simulink model "acceleration_event_simulink"  (R2023b)
settings: Solver=VariableStepAuto  StartTime=0.0  StopTime=10.0  RelTol=1e-3
settings Model: Creator=bglen  LastModifiedBy=bglen
settings DebuggingCC: UnconnectedInputMsg=warning  UnconnectedOutputMsg=warning  UnconnectedLineMsg=warning
settings ModelReferenceCC: EnableRefExpFcnMdlSchedulingChecks=on
settings RTWCC: DLArmComputeVersion=19.05

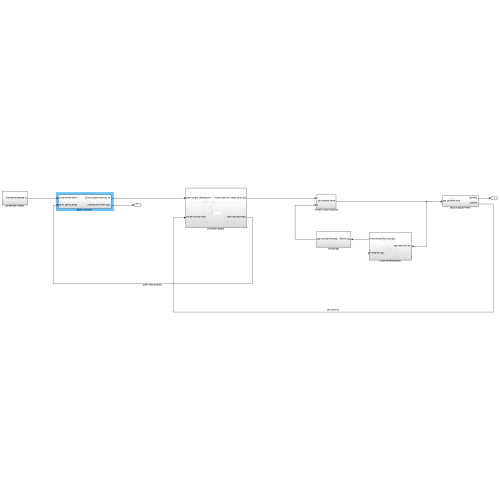
[thumbnail: Simulink's stored preview of the top-level diagram]
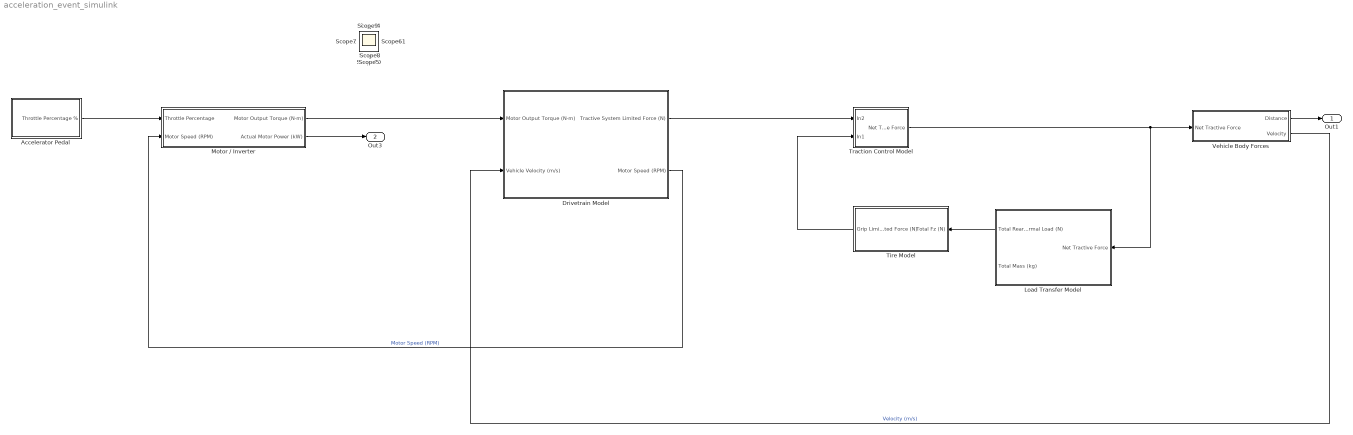
== system acceleration_event_simulink ==
  Accelerator Pedal : Subsystem
  Drivetrain Model : Subsystem
  Load Transfer Model : Subsystem
  Motor / Inverter : Subsystem
  Tire Model : Subsystem
  Traction Control Model : Subsystem
  Vehicle Body Forces : Subsystem
  Out1 : Outport
  Out3 : Outport  Port=2
  Scope{,1..11} (12 alike) : Scope
  wires:
  Load Transfer Model/1(Total Rear Normal Load (N)) -> Tire Model/1(Total Fz (N))
  Vehicle Body Forces/1(Distance) -> Out1/1
  Vehicle Body Forces/2(Velocity) -> Drivetrain Model/2(Vehicle Velocity (m/s))  "Velocity (m/s)"
  Traction Control Model/1(Net Tractive Force) -> Load Transfer Model/1(Net Tractive Force), Vehicle Body Forces/1(Net Tractive Force)
  Tire Model/1(Grip Limited Force (N)) -> Traction Control Model/2(In1)
  Drivetrain Model/1(Tractive System Limited Force (N)) -> Traction Control Model/1(In2)
  Drivetrain Model/2(Motor Speed (RPM)) -> Motor / Inverter/2(Motor Speed (RPM))  "Motor Speed (RPM)"
  Motor / Inverter/1(Motor Output Torque (N-m)) -> Drivetrain Model/1(Motor Output Torque (N-m))
  Motor / Inverter/2(Actual Motor Power (kW)) -> Out3/1
  Accelerator Pedal/1(Throttle Percentage %) -> Motor / Inverter/1(Throttle Percentage)

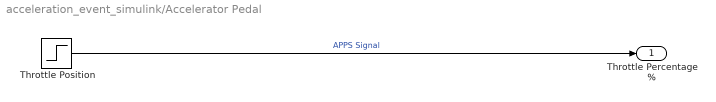
== system acceleration_event_simulink/Accelerator Pedal ==
  Throttle Position : Step  SampleTime=0
  Throttle Percentage % : Outport
  wires:
  Throttle Position/1 -> Throttle Percentage %/1  "APPS Signal"

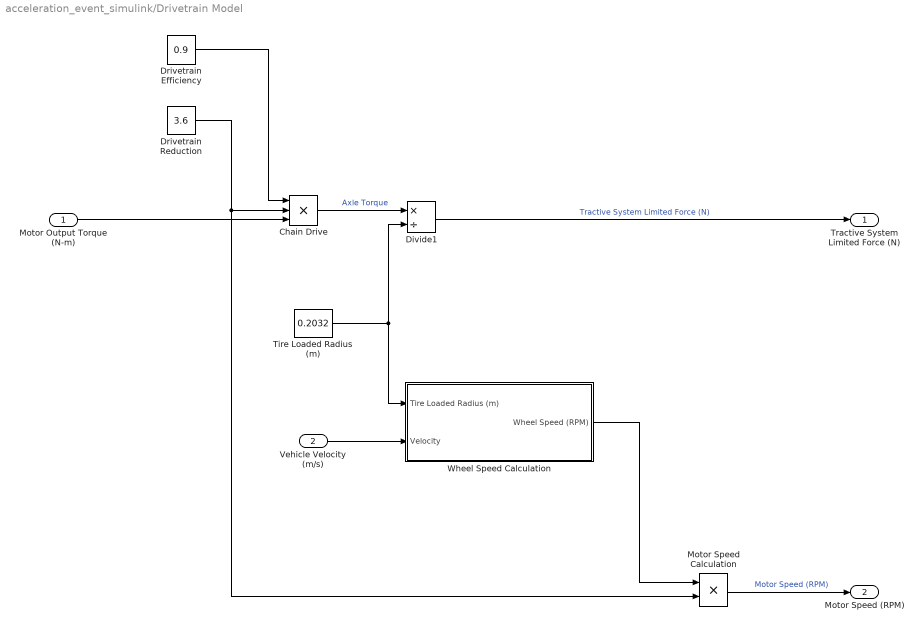
== system acceleration_event_simulink/Drivetrain Model ==
  Motor Output Torque (N-m) : Inport
  Vehicle Velocity (m/s) : Inport  Port=2
  "  Motor Speed Calculation" : Product
  Chain Drive : Product  Inputs=3
  Divide1 : Product  Inputs=*/
  Drivetrain Efficiency : Constant  Value=0.9
  Drivetrain Reduction : Constant  Value=3.6
  Tire Loaded Radius (m) : Constant  Value=0.2032
  Wheel Speed Calculation : Subsystem
  Tractive System Limited Force (N) : Outport
  Motor Speed (RPM) : Outport  Port=2
  wires:
  Divide1/1 -> Tractive System Limited Force (N)/1  "Tractive System Limited Force (N)"
  Tire Loaded Radius (m)/1 -> Wheel Speed Calculation/1(Tire Loaded Radius (m)), Divide1/2
  Chain Drive/1 -> Divide1/1  "Axle Torque"
  Motor Output Torque (N-m)/1 -> Chain Drive/3
  Drivetrain Efficiency/1 -> Chain Drive/1
  Drivetrain Reduction/1 -> "  Motor Speed Calculation"/2, Chain Drive/2
  Vehicle Velocity (m/s)/1 -> Wheel Speed Calculation/2(Velocity)
  Wheel Speed Calculation/1(Wheel Speed (RPM)) -> "  Motor Speed Calculation"/1
  "  Motor Speed Calculation"/1 -> Motor Speed (RPM)/1  "Motor Speed (RPM)"

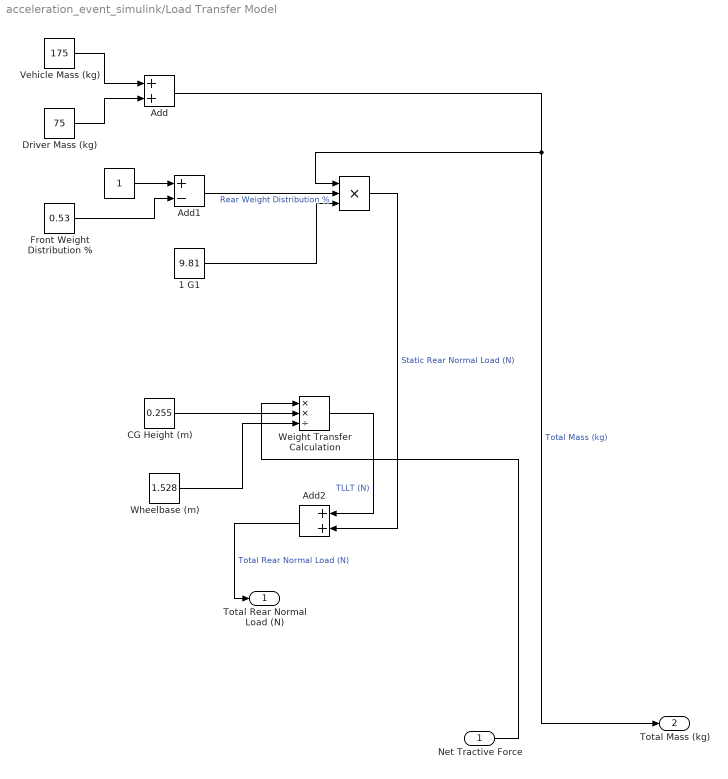
== system acceleration_event_simulink/Load Transfer Model ==
  Net Tractive Force : Inport
  " " : Constant
  "  " : Product  Inputs=3
  "  Weight Transfer Calculation" : Product  Inputs=**/
  1 G1 : Constant  Value=9.81
  Add : Sum
  Add1 : Sum  Inputs=+-
  Add2 : Sum
  CG Height (m) : Constant  Value=0.255
  Driver Mass (kg) : Constant  Value=75
  Front Weight Distribution % : Constant  Value=0.53
  Vehicle Mass (kg) : Constant  Value=175
  Wheelbase (m) : Constant  Value=1.528
  Total Rear Normal Load (N) : Outport
  Total Mass (kg) : Outport  Port=2
  wires:
  Net Tractive Force/1 -> "  Weight Transfer Calculation"/1
  " "/1 -> Add1/1
  "  "/1 -> Add2/2  "Static Rear Normal Load (N)"
  Add1/1 -> "  "/2  "Rear Weight Distribution %"
  Add2/1 -> Total Rear Normal Load (N)/1  "Total Rear Normal Load (N)"
  1 G1/1 -> "  "/3
  Vehicle Mass (kg)/1 -> Add/1
  CG Height (m)/1 -> "  Weight Transfer Calculation"/2
  Front Weight Distribution %/1 -> Add1/2
  Wheelbase (m)/1 -> "  Weight Transfer Calculation"/3
  "  Weight Transfer Calculation"/1 -> Add2/1  "TLLT (N)"
  Add/1 -> Total Mass (kg)/1, "  "/1  "Total Mass (kg)"
  Driver Mass (kg)/1 -> Add/2

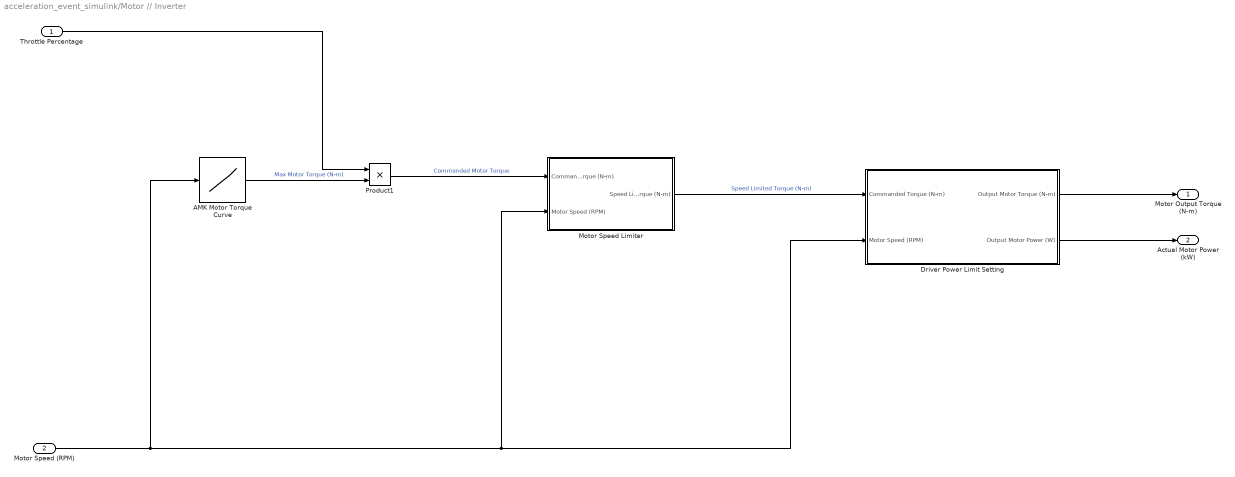
== system acceleration_event_simulink/Motor // Inverter ==
  Throttle Percentage : Inport
  Motor Speed (RPM) : Inport  Port=2
  AMK Motor Torque Curve : Lookup_n-D  NumberOfTableDimensions=1  BreakpointsForDimension1=[0;28.3870968;1447.74194;3179.35484;4740.64516;7267.09677;9055.48387;10872.2581;12178.0645;13029.6774;13994.8387;14846.4516;15612.9032;16095.4839;16805.1613;17571.6129;18423.2258;19274.8387;19785.8065;19984.5161]  Table=[21.31;21.3068182;21.3068182;21.3068182;21.3068182;21.3068182;21.3068182;21.3068182;21.3068182;21.3068182;21.3068182;21.3068182;21.3068182;20.9659091;19.9431818;18.5795455;17.0454545;15.3409091;14.1477273;13.6363636]  InternalRulePriority=Speed  RndMeth=Simplest
  Driver Power Limit Setting : Subsystem
  Motor Speed Limiter : Subsystem
  Product1 : Product
  Motor Output Torque (N-m) : Outport
  Actual Motor Power (kW) : Outport  Port=2
  wires:
  Throttle Percentage/1 -> Product1/1
  Product1/1 -> Motor Speed Limiter/1(Commanded Torque (N-m))  "Commanded Motor Torque"
  Motor Speed (RPM)/1 -> Motor Speed Limiter/2(Motor Speed (RPM)), Driver Power Limit Setting/2(Motor Speed (RPM)), AMK Motor Torque Curve/1
  AMK Motor Torque Curve/1 -> Product1/2  "Max Motor Torque (N-m)"
  Motor Speed Limiter/1(Speed Limited Motor Torque (N-m)) -> Driver Power Limit Setting/1(Commanded Torque (N-m))  "Speed Limited Torque (N-m)"
  Driver Power Limit Setting/1(Output Motor Torque (N-m)) -> Motor Output Torque (N-m)/1
  Driver Power Limit Setting/2(Output Motor Power (W)) -> Actual Motor Power (kW)/1

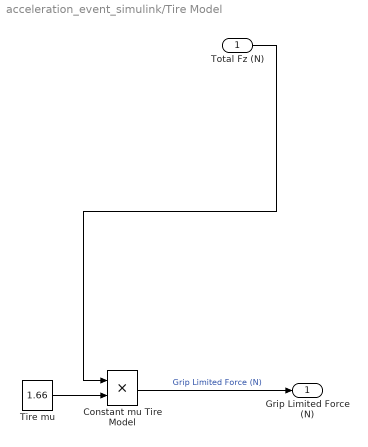
== system acceleration_event_simulink/Tire Model ==
  Total Fz (N) : Inport
  Constant mu Tire Model : Product
  Tire mu : Constant  Value=1.66
  Grip Limited Force (N) : Outport
  wires:
  Total Fz (N)/1 -> Constant mu Tire Model/1
  Constant mu Tire Model/1 -> Grip Limited Force (N)/1  "Grip Limited Force (N)"
  Tire mu/1 -> Constant mu Tire Model/2

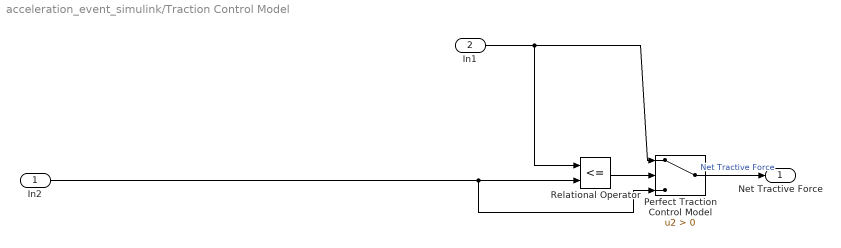
== system acceleration_event_simulink/Traction Control Model ==
  In2 : Inport
  In1 : Inport  Port=2
  Perfect Traction Control Model : Switch  Criteria=u2 > Threshold  SaturateOnIntegerOverflow=off  InputSameDT=off
  Relational Operator : RelationalOperator  Operator=<=  OutDataTypeStr=boolean  RndMeth=Simplest  InputSameDT=off
  Net Tractive Force : Outport
  wires:
  Perfect Traction Control Model/1 -> Net Tractive Force/1  "Net Tractive Force"
  Relational Operator/1 -> Perfect Traction Control Model/2
  In1/1 -> Relational Operator/1, Perfect Traction Control Model/1
  In2/1 -> Perfect Traction Control Model/3, Relational Operator/2

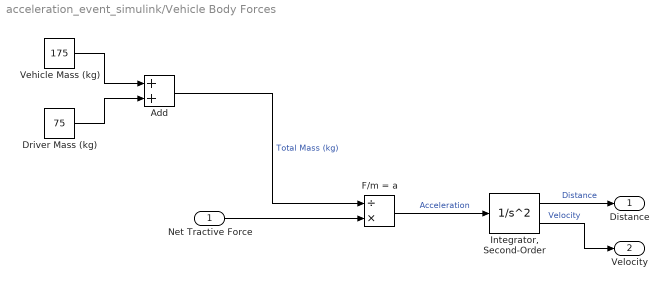
== system acceleration_event_simulink/Vehicle Body Forces ==
  Net Tractive Force : Inport
  Add : Sum
  Driver Mass (kg) : Constant  Value=75
  F/m = a : Product  Inputs=/*
  "Integrator, Second-Order" : SecondOrderIntegrator  LimitX=on  UpperLimitX=75
  Vehicle Mass (kg) : Constant  Value=175
  Distance : Outport
  Velocity : Outport  Port=2
  wires:
  "Integrator, Second-Order"/2 -> Velocity/1  "Velocity"
  Net Tractive Force/1 -> F/m = a/2
  "Integrator, Second-Order"/1 -> Distance/1  "Distance"
  F/m = a/1 -> "Integrator, Second-Order"/1  "Acceleration"
  Driver Mass (kg)/1 -> Add/2
  Vehicle Mass (kg)/1 -> Add/1
  Add/1 -> F/m = a/1  "Total Mass (kg)"

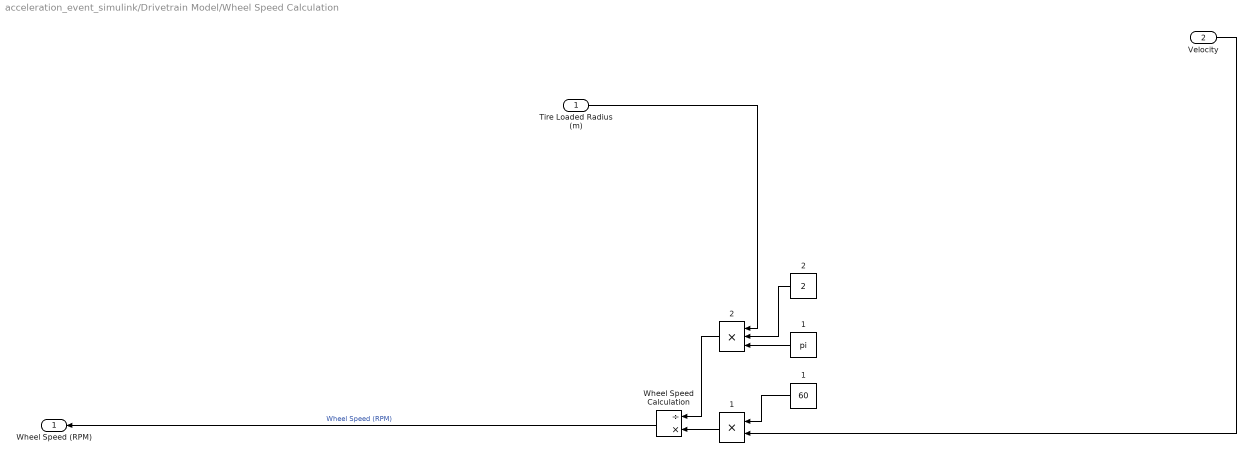
== system acceleration_event_simulink/Drivetrain Model/Wheel Speed Calculation ==
  Tire Loaded Radius (m) : Inport
  Velocity : Inport  Port=2
  "  1" : Product
  "  2" : Product  Inputs=3
  " 1" : Constant  Value=60
  1 : Constant  Value=pi
  2 : Constant  Value=2
  Wheel Speed Calculation : Product  Inputs=/*
  Wheel Speed (RPM) : Outport
  wires:
  Tire Loaded Radius (m)/1 -> "  2"/1
  Velocity/1 -> "  1"/2
  " 1"/1 -> "  1"/1
  "  2"/1 -> Wheel Speed Calculation/1
  1/1 -> "  2"/3
  "  1"/1 -> Wheel Speed Calculation/2
  Wheel Speed Calculation/1 -> Wheel Speed (RPM)/1  "Wheel Speed (RPM)"
  2/1 -> "  2"/2

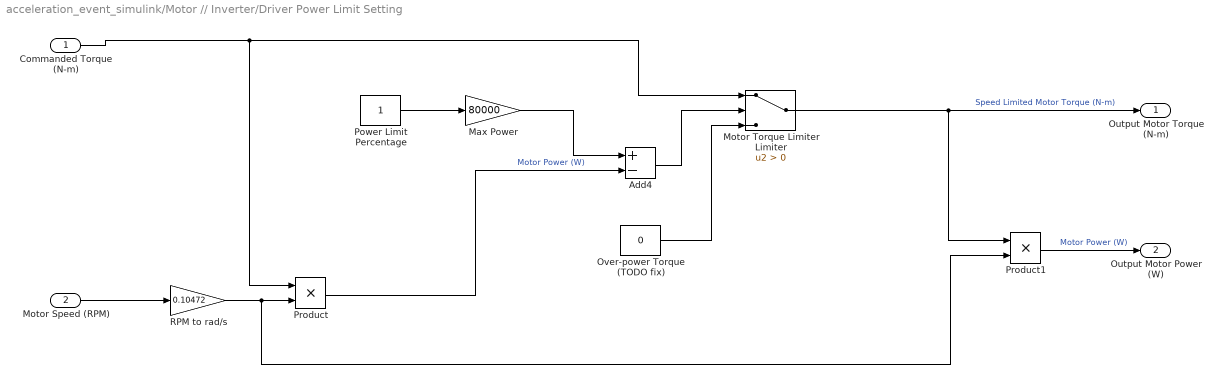
== system acceleration_event_simulink/Motor // Inverter/Driver Power Limit Setting ==
  Commanded Torque (N-m) : Inport
  Motor Speed (RPM) : Inport  Port=2
  Add4 : Sum  Inputs=+-
  Max Power : Gain  Gain=80000
  Motor Torque Limiter Limiter : Switch  Criteria=u2 > Threshold  SaturateOnIntegerOverflow=off  InputSameDT=off
  Over-power Torque (TODO fix) : Constant  Value=0
  Power Limit Percentage : Constant
  Product : Product
  Product1 : Product
  RPM to rad/s : Gain  Gain=0.10472
  Output Motor Torque (N-m) : Outport
  Output Motor Power (W) : Outport  Port=2
  wires:
  Add4/1 -> Motor Torque Limiter Limiter/2
  Commanded Torque (N-m)/1 -> Motor Torque Limiter Limiter/1, Product/1
  Motor Torque Limiter Limiter/1 -> Product1/1, Output Motor Torque (N-m)/1  "Speed Limited Motor Torque (N-m)"
  Over-power Torque (TODO fix)/1 -> Motor Torque Limiter Limiter/3
  Motor Speed (RPM)/1 -> RPM to rad/s/1
  Power Limit Percentage/1 -> Max Power/1
  Product/1 -> Add4/2  "Motor Power (W)"
  Max Power/1 -> Add4/1
  RPM to rad/s/1 -> Product1/2, Product/2
  Product1/1 -> Output Motor Power (W)/1  "Motor Power (W)"

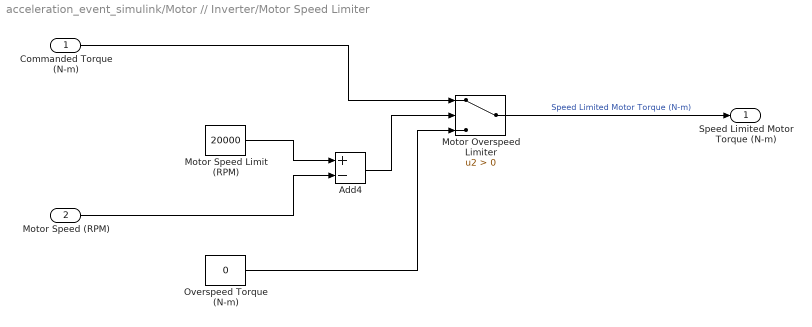
== system acceleration_event_simulink/Motor // Inverter/Motor Speed Limiter ==
  Commanded Torque (N-m) : Inport
  Motor Speed (RPM) : Inport  Port=2
  Add4 : Sum  Inputs=+-
  Motor Overspeed Limiter : Switch  Criteria=u2 > Threshold  SaturateOnIntegerOverflow=off  InputSameDT=off
  Motor Speed Limit (RPM) : Constant  Value=20000
  Overspeed Torque (N-m) : Constant  Value=0
  Speed Limited Motor Torque (N-m) : Outport
  wires:
  Motor Speed (RPM)/1 -> Add4/2
  Add4/1 -> Motor Overspeed Limiter/2
  Commanded Torque (N-m)/1 -> Motor Overspeed Limiter/1
  Motor Speed Limit (RPM)/1 -> Add4/1
  Motor Overspeed Limiter/1 -> Speed Limited Motor Torque (N-m)/1  "Speed Limited Motor Torque (N-m)"
  Overspeed Torque (N-m)/1 -> Motor Overspeed Limiter/3
